simulink model "uas_main"  (R2021a)
settings: Solver=FixedStepAuto  StartTime=0.0  StopTime=5  FixedStep=sample_time  RelTol=1e-3
model workspace: external: MAT-File (data not in the file)
values from neighbouring files (symbols this model uses):
  arm_length = 0.17    [uas_parameters.m]    (also in uas_parameters.mat)
  drag_coefficient = 0.47    [uas_parameters.m]    (also in uas_parameters.mat)
  g = 9.80665    [uas_parameters.m]    (also in uas_parameters.mat)
  inertia_xx = 0.007    [uas_parameters.m]    (also in uas_parameters.mat)
  inertia_yy = 0.007    [uas_parameters.m]    (also in uas_parameters.mat)
  inertia_zz = 0.012    [uas_parameters.m]    (also in uas_parameters.mat)
  mass_drone = 0.68    [uas_parameters.m]    (also in uas_parameters.mat)
  mass_total = mass_drone + mass_rod + mass_tip    (= 0.68)    [uas_parameters.m]    (also in uas_parameters.mat)
  max_rot_velocity = 838    [uas_parameters.m]    (also in uas_parameters.mat)
  mix_matrix = inv(motor_constant * allocation_matrix)    [uas_parameters.m]    (also in uas_parameters.mat = [29244.6230836 29244.6230836 29244.6230836 29244.6230836 -5.)
  moment_constant = 0.016    [uas_parameters.m]    (also in uas_parameters.mat)
  motor_constant = 8.54858e-06    [uas_parameters.m]    (also in uas_parameters.mat)
  poly_traj = uas_minimum_snap(knots, order, waypoints, corridors, make_plots)    [uas_trajectory.m]
  publish_rate = 1 * sample_time    (= 0.04)    [uas_parameters.m]    (also in uas_parameters.mat)
  reference_area = pi * 75e-3^2    (= 0.0176714586764)    [uas_parameters.m]    (also in uas_parameters.mat)
  rotor_offset_top = 0.01    [uas_parameters.m]    (also in uas_parameters.mat)
  route = [0 0 1 ; 9 0 1 ; 9 5 1; 7 5 1; 7 7 1; 5 7 1; 5 5 1; 3 5 1]    [uas_parameters.m]    (also in uas_parameters.mat = [0  0  1; 9  0  1; 9  9  1])
  sample_time = 4e-2    (= 0.04)    [uas_parameters.m]    (also in uas_parameters.mat)
  x0 = 36    [uas_parameters.m]    (also in uas_parameters.mat)
  y0 = 80    [uas_parameters.m]    (also in uas_parameters.mat)
  z0 = 1    [uas_parameters.m]    (also in uas_parameters.mat)
undefined symbols (not defined in the file or in its folder): Angular, Linear, Pose, Position, quat2rotm, X, Y, Z
libraries: nesl_utility x32, sm_lib x25, robotlib x9, simulink x1, sim3dlib x1, uavsim3dlib x1, vrlib x1
(part 1 of 2)
settings Model: EnablePacing=on  Creator=david  LastModifiedBy=emilm
settings SolverCC: AlgebraicLoopSolver=TrustRegion
settings DataIOCC: LimitDataPoints=on  MaxDataPoints=10000
settings OptimizationCC: EnhancedBackFolding=on  PassReuseOutputArgsThreshold=0  ZeroExternalMemoryAtStartup=off  ZeroInternalMemoryAtStartup=off  MaxStackSize=64  OptimizeBlockOrder=speed  DifferentSizesBufferReuse=on  OptimizationCustomize=off
settings DebuggingCC: ParameterTunabilityLossMsg=error  AllowSymbolicDim=off  SFUnexpectedBacktrackingDiag=warning  SFNoUnconditionalDefaultTransitionDiag=warning  SFExecutionAtInitializationDiag=none  SFMachineParentedDataDiag=warning  UnderSpecifiedDimensionMsg=warning  ArithmeticOperatorsInVariantConditions=warning
settings HardwareCC: ProdBitPerPointer=32  ProdBitPerSizeT=32  ProdBitPerPtrDiffT=32  ProdLargestAtomicFloat=None  ProdIntDivRoundTo=Undefined  ProdEndianess=Unspecified  ProdWordSize=32  ProdHWDeviceType=Generic->Unspecified (assume 32-bit Generic)  UseEmbeddedCoderFeatures=off
settings SFSimCC: SimUseLocalCustomCode=off  MATLABDynamicMemAlloc=off  CustomCodeUndefinedFunction=UseInterfaceOnly  SimTargetLang=C++
settings RTWCC: SystemTargetFile=ert.tlc  HardwareBoard=Robot Operating System (ROS)  TLCOptions="-aInlineSetEventsForThisBaseRateFcn=TLC_FALSE -aSuppressMultiTaskScheduler=TLC_FALSE  -aRateBasedStepFcn=0"  TemplateMakefile=ert_default_tmf  RTWUseLocalCustomCode=off  Toolchain=Catkin  TargetLang=C++
settings CodeAppCC: ForceParamTrailComments=on  OperatorAnnotations=on
settings ERTTargetCC: ERTCustomFileBanners=off  CodeInterfacePackaging=C++ class  SupportContinuousTime=on  SupportNonInlinedSFcns=on  RemoveResetFunc=off  ModelStepFunctionPrototypeControlCompliant=off  RootIOFormat=Structure reference
settings ConfigComp: CovMetricSettings=dw  CovSaveCumulativeToWorkspaceVar=on  CovSaveSingleToWorkspaceVar=on  CovExternalEMLEnable=off  CovSFcnEnable=off
settings SimscapeCC: SimscapeLogType=all  SimscapeLogSimulationStatistics=on  SimscapeLogDataHistory=10000
settings ExplorerConfigSet: InternalSimMechanicsExplorerSettings="<ExplorerConfiguration><canonicalview>default</canonicalview><AnimationSetting><BasePlaybackSpeed>1.0</BasePlaybackSpeed><PlaybackSpeedFactor>1.0</PlaybackSpeedFactor></AnimationSetting><TilePanel><TileInfo><Tiles Columns=\"1\" Count=\"1\" Rows=\"1\"><Column Weight=\"1\"/><Row Weight=\"1\"/><Tile Height=\"1\" Width=\"1\" X=\"0\" Y=\"0\"/></Tiles></TileInfo><SceneInfo><SceneViewer><BGColor><R>0.400000005960464478</R><G>0.400000005960464478</G><B>0.400000005960464478</B></BGColor><Camera><DoPerspective>off</DoPerspective><Position><X>7.41918867546502359</X><Y>0.562842449888731333</Y><Z>8.36768126399918444</Z></Position><Center><X>4.24878770726833288</X><Y>4.27540210027623324</Y><Z>0.996100590645515815</Z></Center><Up><X>-0.578313069199200891</X><Y>0.601173295476169489</Y><Z>0.551493121262380703</Z></Up><ViewLimDist>1</ViewLimDist><YLim>5.48746925830841104</YLim><XLim>8.41878250057976274</XLim></Camera></SceneViewer></SceneInfo></TilePanel><MechEditorPanel><Cameras/><GfxPanelCameraMap/><VideoCreator><PlaybackSpeedRatio>1.0</PlaybackSpeedRatio><FrameRate>30</FrameRate><VideoFormat>Motion JPEG AVI</VideoFormat><FrameSize>auto</FrameSize></VideoCreator></MechEditorPanel></ExplorerConfiguration>"

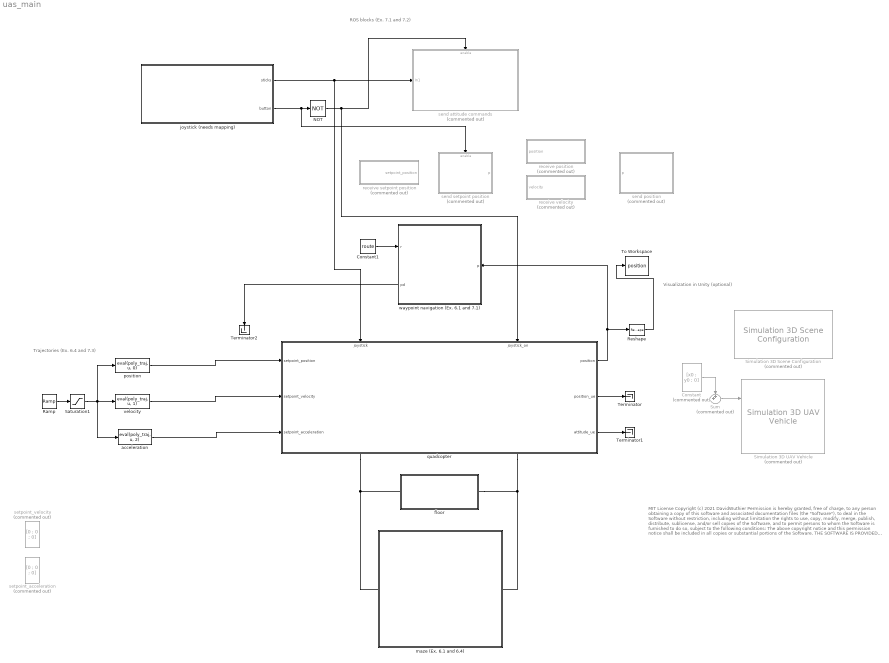
== system uas_main ==
  note: MIT License
      |
      | Copyright (c) 2021 DavidWuthier
      |
      | Permission is hereby granted, free of charge, to any person obtaining a copy
      | of this software and associated documentation files (the "Software"), to deal
      | in the Software without restriction, including without limitation the rights
      | to use, copy, modify, merge, publish, distribute, sublicense, and/or sell
      | copies of the Software, and to permit persons to whom the Software is
      | furnished to do so, subject to the following conditions:
      |
      | The above copyright notice and this permission notice shall be included in all
      | copies or substantial portions of the Software.
      |
      | THE SOFTWARE IS PROVIDED "AS IS", WITHOUT WARRANTY OF ANY KIND, EXPRESS OR
      | IMPLIED, INCLUDING BUT NOT LIMITED TO THE WARRANTIES OF MERCHANTABILITY,
      | FITNESS FOR A PARTICULAR PURPOSE AND NONINFRINGEMENT. IN NO EVENT SHALL THE
      | AUTHORS OR COPYRIGHT HOLDERS BE LIABLE FOR ANY CLAIM, DAMAGES OR OTHER
      | LIABILITY, WHETHER IN AN ACTION OF CONTRACT, TORT OR OTHERWISE, ARISING FROM,
      | OUT OF OR IN CONNECTION WITH THE SOFTWARE OR THE USE OR OTHER DEALINGS IN THE
      | SOFTWARE.
  note: Visualization in Unity (optional)
  note: Trajectories (Ex. 6.4 and 7.3)
  note: ROS blocks (Ex. 7.1 and 7.2)
  Constant : Constant  Commented=on  Value=[x0 ; y0 ; 0]  VectorParams1D=off
  Constant1 : Constant  Value=route
  NOT : Logic  Operator=NOT  IconShape=distinctive  AllPortsSameDT=off  OutDataTypeStr=boolean
  Ramp : simulink/Sources/Ramp  slope=1  start=0  InitialOutput=0
  Reshape : Reshape  OutputDimensions=[3,:]
  Saturation1 : Saturate  UpperLimit=knots(end)  LowerLimit=0
  Simulation 3D Scene Configuration : sim3dlib/Simulation 3D Scene Configuration  Priority=0  Commented=on  ProjectFormat=Default Scenes  SceneDesc=US city block  ProjectName=C:\Program Files\MATLAB\R2021a\toolbox\shared\sim3d_projects\automotive_project\UE4\WindowsNoEditor\VehicleSimulation.exe  ScenePath=/Game/Maps/USCityBlock  vehTagList={'Scene Origin';'SimulinkVehicle1'}  vehTag=SimulinkVehicle1  OpVisEn=off  Ts=sample_time  EnableWindow=on  EnableWeather=off  SunAltitude=40.0  SunAzimuth=90  clouds=10  wind=1  fog=0  rain=0  sensorTag=MainCamera1  sensorId=1  sensorName=MainCamera1  mountLoc=Origin  offsetFlag=off  tmountOffset=[0, 0, 0]  rmountOffset=[0, 0, 0]  HorizontalResolution=1280  VerticalResolution=720  HorizontalFOV=60  mountPoint=[0 0 0]  mountOrientation=[0 0 0]  aMode=4  ID=1
      settings: SourceProductBaseCode=DR,UV,VE
  Simulation 3D UAV Vehicle : uavsim3dlib/Simulation 3D UAV Vehicle  Commented=on  Mesh=Quadrotor  Color=Black  ActorName=SimulinkVehicle1  InitialTranslation=[x0 y0 z0]  InitialRotation=[0 0 0]  SampleTime=-1  ActorType=SimulinkVehicle  ID=1  aMode=4  ActorTag=SimulinkVehicle1
      settings: SourceProductBaseCode=UV
  Sum : Sum  Commented=on  Inputs=++|
  Terminator : Terminator
  Terminator1 : Terminator
  Terminator2 : Terminator
  To Workspace : ToWorkspace  VariableName=position  SampleTime=-1
  acceleration : MATLABFcn  MATLABFcn=eval(poly_traj, u, 2)  OutputDimensions=[3 1]  Output1D=off
  floor : Subsystem
  joystick (needs mapping) : Subsystem
  maze (Ex. 6.1 and 6.4) : Subsystem
      mask Display: image('$imagefile'); % Use "Edit Image" on toolstrip to change.
  position : MATLABFcn  MATLABFcn=eval(poly_traj, u, 0)  OutputDimensions=[3 1]  Output1D=off
  quadcopter : Subsystem
      settings: PortSchema="{\"entries\":[{\"content\":{\"sides\":[{\"content\":{\"connectorIds\":[\"In1\",\"In2\",\"In3\"]},\"type\":\"ConnectorPlacement.EquallySpacedRectSide\",\"uuid\":\"ed16c4a7-5f5f-48d5-8471-b227eef37b0b\"},{\"content\":{\"connectorIds\":[\"Out1\",\"Out2\",\"Out3\"],\"side\":\"RIGHT\"},\"type\":\"ConnectorPlacement.EquallySpacedRectSide\",\"uuid\":\"303ea24f-0a15-469a-b5d8-cc8b33d29b5f\"},{\"content\":{\"connectorIds\":[\"In4\",\"In5\"],\"side\":\"TOP\"},\"type\":\"ConnectorPlacement.EquallySpacedRectSide\",\"uuid\":\"d3970502-0872-434b-b7c5-387e72ad4178\"},{\"content\":{\"connectorIds\":[\"RConn1\",\"RConn2\"],\"side\":\"BOTTOM\"},\"type\":\"ConnectorPlacement.EquallySpacedRectSide\",\"uuid\":\"dd808c8e-2f91-44fb-8d51-5dec3bd81dd9\"}]},\"type\":\"ConnectorPlacement.EquallySpacedConnector\",\"uuid\":\"aacf4a84-08b7-4fd3-a02a-51c4e2a4df71\"}],\"packageUris\":[\"http://schema.mathworks.com/mf0/Connector/R2020b\"],\"version\":\"1.0\"}"
  receive position : Subsystem  Commented=on
  receive setpoint position : Subsystem  Commented=on
  receive velocity : Subsystem  Commented=on
  send attitude commands : Subsystem  Commented=on
  send position : Subsystem  Commented=on
  send setpoint position : Subsystem  Commented=on
  setpoint_acceleration : Constant  Commented=on  Value=[0 ; 0 ; 0]  VectorParams1D=off
  setpoint_velocity : Constant  Commented=on  Value=[0 ; 0 ; 0]  VectorParams1D=off
  velocity : MATLABFcn  MATLABFcn=eval(poly_traj, u, 1)  OutputDimensions=[3 1]  Output1D=off
  waypoint navigation (Ex. 6.1 and 7.1) : Stateflow chart  TreatAsAtomicUnit=on
      settings: PortSchema="{\"entries\":[{\"content\":{\"sides\":[{\"content\":{\"connectorIds\":[\"In1\",\"Out1\"]},\"type\":\"ConnectorPlacement.EquallySpacedRectSide\",\"uuid\":\"7c2fff0d-1179-4786-9432-1971d7acd904\"},{\"content\":{\"connectorIds\":[\"In2\"],\"side\":\"RIGHT\"},\"type\":\"ConnectorPlacement.EquallySpacedRectSide\",\"uuid\":\"377a8206-b310-41c0-9a17-faf5318c89cb\"},{\"content\":{\"connectorIds\":[],\"side\":\"TOP\"},\"type\":\"ConnectorPlacement.EquallySpacedRectSide\",\"uuid\":\"b953090a-ffdb-4e30-a5fe-7bef9655f1cf\"},{\"content\":{\"connectorIds\":[],\"side\":\"BOTTOM\"},\"type\":\"ConnectorPlacement.EquallySpacedRectSide\",\"uuid\":\"03dc7a24-529e-4020-b953-d1c4751c5c80\"}]},\"type\":\"ConnectorPlacement.EquallySpacedConnector\",\"uuid\":\"03bac9f4-6480-492d-9af3-57aec4db8fd8\"}],\"packageUris\":[\"http://schema.mathworks.com/mf0/Connector/R2020b\"],\"version\":\"1.0\"}"
  wires:
  Sum/1 -> Simulation 3D UAV Vehicle/1
  Constant/1 -> Sum/1
  Constant1/1 -> waypoint navigation (Ex. 6.1 and 7.1)/1(r)
  Saturation1/1 -> acceleration/1, position/1, velocity/1
  Ramp/1 -> Saturation1/1
  NOT/1 -> quadcopter/5(joystick_on), send attitude commands/Enable
  joystick (needs mapping)/1(sticks) -> send attitude commands/1(In1), quadcopter/4(joystick)
  joystick (needs mapping)/2(button) -> NOT/1, send setpoint position/Enable
  quadcopter/1(position) -> Reshape/1, waypoint navigation (Ex. 6.1 and 7.1)/2(p)
  quadcopter/2(position_ue) -> Terminator/1
  quadcopter/3(attitude_ue) -> Terminator1/1
  Reshape/1 -> To Workspace/1
  waypoint navigation (Ex. 6.1 and 7.1)/1(pd) -> Terminator2/1
  position/1 -> quadcopter/1(setpoint_position)
  velocity/1 -> quadcopter/2(setpoint_velocity)
  acceleration/1 -> quadcopter/3(setpoint_acceleration)
  connections:
  floor/LConn1 -- quadcopter/RConn1 -- maze (Ex. 6.1 and 6.4)/LConn1
  floor/RConn1 -- quadcopter/RConn2 -- maze (Ex. 6.1 and 6.4)/RConn1

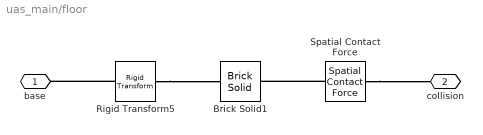
== system uas_main/floor ==
  Brick Solid1 : sm_lib/Body Elements/Brick Solid  GraphicAmbientColor=[0.15 0.15 0.15 1.0]  BasedOnType=Density  BrickDimensions=[3 3 0.1]  BrickDimensionUnits=m  CenterOfMass=[0 0 0]  CenterOfMassUnits=m  GraphicDiffuseColor=[0.4 0.4 0.4]  Density=0  DensityUnits=kg/m^3  DoExposeReferenceFrame=on  GraphicEmissiveColor=[0.0 0.0 0.0 1.0]  ExportEntireGeometry=on  SerializedFrames=<Frames/>  MarkerShape=Sphere  MarkerSize=10  GraphicType=FromGeometry  InertiaType=CalculateFromGeometry  Mass=1  MassUnits=kg  MomentsOfInertia=[1 1 1]  MomentsOfInertiaUnits=kg*m^2  GraphicOpacity=1  ProductsOfInertia=[0 0 0]  ProductsOfInertiaUnits=kg*m^2  GraphicShininess=75  GraphicSpecularColor=[0.5 0.5 0.5 1.0]  GraphicVisPropType=SimpleVisualProperties
  Rigid Transform5 : sm_lib/Frames and Transforms/Rigid Transform  TranslationMethod=StandardAxis  TranslationStandardOffset=0.05  TranslationLengthUnit=m  TranslationStandardAxis=-Z  TranslationCartesianOffset=[0 0 0]  TranslationROffset=0  TranslationROffsetUnits=m  TranslationZOffset=0  TranslationZOffsetUnits=m  TranslationThetaOffset=0  TranslationThetaOffsetUnits=deg  RotationMethod=None  RotationAngleUnits=deg  RotationStandardAxis=+Z  RotationAngle=0.0  RotationArbitraryAxis=[0 0 1]  FollAlignAxisA=+X  BaseAlignAxisA=+Y  FollAlignAxisB=+Y  BaseAlignAxisB=+Z  RotationSequenceAxes=FollowerAxes  RotationSequence=XYX  RotationSequenceAngles=[0 0 0]  RotationSequenceAnglesUnits=deg  RotationMatrix=[1 0 0; 0 1 0; 0 0 1]
  Spatial Contact Force : sm_lib/Forces and Torques/Spatial Contact Force  CoefficientOfDynamicFriction=0.3  CoefficientOfStaticFriction=0.5  SenseContactBaseRotation=off  SenseContactBaseTranslation=off  NormalDamping=critical_damping_wall  NormalDampingUnits=N/(m/s)  SenseContactFollowerRotation=off  SenseContactFollowerTranslation=off  SenseContactSignal=off  NormalStiffness=stiffness_wall  NormalStiffnessUnits=N/m  FrictionalCriticalVelocity=1e-3  FrictionalCriticalVelocityUnits=m/s  ZeroCrossDetectContactStartAndEnd=off  FrictionType=SmoothStickSlip  SenseFrictionalForceMagnitude=off  SenseNormalForceMagnitude=off  NormalForceType=SmoothSpringDamper  SenseNormalVelocity=off  SenseSeparationDistance=off  SenseTangentialVelocity=off  SenseTangentialVelocityMagnitude=off  NormalTransitionRegionWidth=1e-4  NormalTransitionRegionWidthUnits=m
  base : PMIOPort  Side=Left
  collision : PMIOPort  Port=2  Side=Right
  connections:
  Rigid Transform5/RConn1 -- Brick Solid1/RConn1
  Rigid Transform5/LConn1 -- base/RConn1
  Spatial Contact Force/RConn1 -- Brick Solid1/LConn1
  Spatial Contact Force/LConn1 -- collision/RConn1

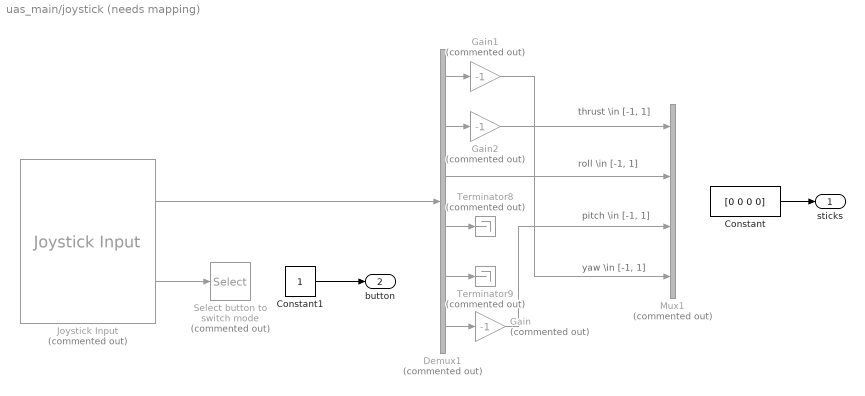
== system uas_main/joystick (needs mapping) ==
  note: thrust \in [-1, 1]
  note: roll \in [-1, 1]
  note: pitch \in [-1, 1]
  note: yaw \in [-1, 1]
  Constant : Constant  Value=[0 0 0 0]
  Constant1 : Constant
  Demux1 : Demux  Commented=on  Outputs=6
  Gain : Gain  Commented=on  Gain=-1
  Gain1 : Gain  Commented=on  Gain=-1
  Gain2 : Gain  Commented=on  Gain=-1
  Joystick Input : vrlib/Joystick Input  Commented=on  joyid=1  adjustports=on  forcefeed=off
  Mux1 : Mux  Commented=on
  Select button to switch mode : Selector  Commented=on  InputPortWidth=15  IndexOptions=Index vector (dialog)  Indices=8  OutputSizes=1
  Terminator8 : Terminator  Commented=on
  Terminator9 : Terminator  Commented=on
  sticks : Outport
  button : Outport  Port=2
  wires:
  Gain1/1 -> Mux1/4
  Joystick Input/1 -> Demux1/1
  Gain2/1 -> Mux1/1
  Demux1/1 -> Gain1/1
  Joystick Input/2 -> Select button to switch mode/1
  Demux1/6 -> Gain/1
  Demux1/5 -> Terminator9/1
  Demux1/3 -> Mux1/2
  Demux1/2 -> Gain2/1
  Demux1/4 -> Terminator8/1
  Gain/1 -> Mux1/3
  Constant/1 -> sticks/1
  Constant1/1 -> button/1

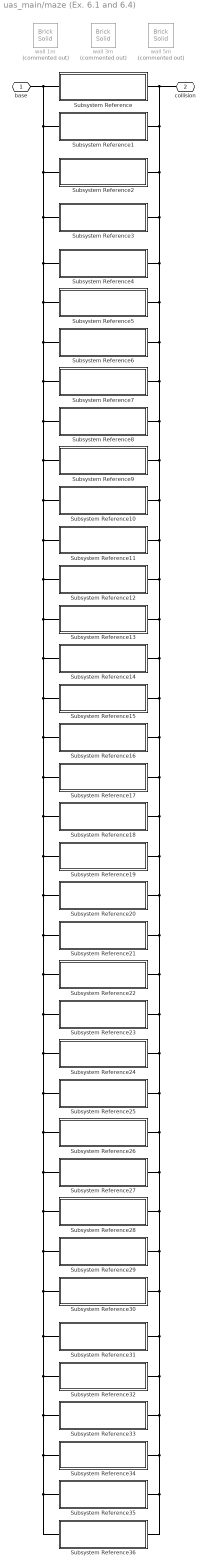
== system uas_main/maze (Ex. 6.1 and 6.4) ==
  Subsystem Reference : Subsystem  ReferencedSubsystem=uas_wall  l=5  x=-1  y=1.5  yaw=0
  Subsystem Reference1 : Subsystem  ReferencedSubsystem=uas_wall  l=5  x=-1  y=7.5  yaw=0
  Subsystem Reference10 : Subsystem  ReferencedSubsystem=uas_wall  l=5  x=7.5  y=10  yaw=pi/2
  Subsystem Reference11 : Subsystem  ReferencedSubsystem=uas_wall  l=5  x=5  y=10  yaw=pi/2
  Subsystem Reference12 : Subsystem  ReferencedSubsystem=uas_wall  l=5  x=1.5  y=1  yaw=pi/2
  Subsystem Reference13 : Subsystem  ReferencedSubsystem=uas_wall  l=3  x=4.5  y=1  yaw=pi/2
  Subsystem Reference14 : Subsystem  ReferencedSubsystem=uas_wall  l=3  x=8  y=2.5  yaw=0
  Subsystem Reference15 : Subsystem  ReferencedSubsystem=uas_wall  l=1  x=6  y=4.5  yaw=0
  Subsystem Reference16 : Subsystem  ReferencedSubsystem=uas_wall  l=1  x=6  y=1.5  yaw=0
  Subsystem Reference17 : Subsystem  ReferencedSubsystem=uas_wall  l=1  x=2  y=1.5  yaw=0
  Subsystem Reference18 : Subsystem  ReferencedSubsystem=uas_wall  l=1  x=0  y=2.5  yaw=0
  Subsystem Reference19 : Subsystem  ReferencedSubsystem=uas_wall  l=5  x=5.5  y=4  yaw=pi/2
  Subsystem Reference2 : Subsystem  ReferencedSubsystem=uas_wall  l=5  x=-1  y=5  yaw=0
  Subsystem Reference20 : Subsystem  ReferencedSubsystem=uas_wall  l=1  x=4  y=3.5  yaw=0
  Subsystem Reference21 : Subsystem  ReferencedSubsystem=uas_wall  l=1  x=2.5  y=4  yaw=pi/2
  Subsystem Reference22 : Subsystem  ReferencedSubsystem=uas_wall  l=1  x=0.5  y=2  yaw=pi/2
  Subsystem Reference23 : Subsystem  ReferencedSubsystem=uas_wall  l=1  x=1.5  y=2  yaw=pi/2
  Subsystem Reference24 : Subsystem  ReferencedSubsystem=uas_wall  l=1  x=-0.5  y=3  yaw=pi/2
  Subsystem Reference25 : Subsystem  ReferencedSubsystem=uas_wall  l=1  x=2  y=4.5  yaw=0
  Subsystem Reference26 : Subsystem  ReferencedSubsystem=uas_wall  l=1  x=1.5  y=5  yaw=pi/2
  Subsystem Reference27 : Subsystem  ReferencedSubsystem=uas_wall  l=1  x=0.5  y=7  yaw=pi/2
  Subsystem Reference28 : Subsystem  ReferencedSubsystem=uas_wall  l=1  x=1  y=7.5  yaw=0
  Subsystem Reference29 : Subsystem  ReferencedSubsystem=uas_wall  l=2  x=8  y=7  yaw=0
  Subsystem Reference3 : Subsystem  ReferencedSubsystem=uas_wall  l=5  x=10  y=1.5  yaw=0
  Subsystem Reference30 : Subsystem  ReferencedSubsystem=uas_wall  l=1  x=-0.5  y=7  yaw=pi/2
  Subsystem Reference31 : Subsystem  ReferencedSubsystem=uas_wall  l=1  x=6  y=5.5  yaw=0
  Subsystem Reference32 : Subsystem  ReferencedSubsystem=uas_wall  l=5  x=5.5  y=8  yaw=pi/2
  Subsystem Reference33 : Subsystem  ReferencedSubsystem=uas_wall  l=1  x=3.5  y=7  yaw=pi/2
  Subsystem Reference34 : Subsystem  ReferencedSubsystem=uas_wall  l=1  x=3  y=7.5  yaw=0
  Subsystem Reference35 : Subsystem  ReferencedSubsystem=uas_wall  l=1  x=4  y=6.5  yaw=0
  Subsystem Reference36 : Subsystem  ReferencedSubsystem=uas_wall  l=1  x=4  y=7.5  yaw=0
  Subsystem Reference4 : Subsystem  ReferencedSubsystem=uas_wall  l=5  x=10  y=7.5  yaw=0
  Subsystem Reference5 : Subsystem  ReferencedSubsystem=uas_wall  l=5  x=10  y=5  yaw=0
  Subsystem Reference6 : Subsystem  ReferencedSubsystem=uas_wall  l=5  x=1.5  y=-1  yaw=pi/2
  Subsystem Reference7 : Subsystem  ReferencedSubsystem=uas_wall  l=5  x=7.5  y=-1  yaw=pi/2
  Subsystem Reference8 : Subsystem  ReferencedSubsystem=uas_wall  l=5  x=5  y=-1  yaw=pi/2
  Subsystem Reference9 : Subsystem  ReferencedSubsystem=uas_wall  l=5  x=1.5  y=10  yaw=pi/2
  wall 1m : sm_lib/Body Elements/Brick Solid  Commented=on  GraphicAmbientColor=[0.15 0.15 0.15 1.0]  BasedOnType=Density  BrickDimensions=[0.1 1 2]  BrickDimensionUnits=m  CenterOfMass=[0 0 0]  CenterOfMassUnits=m  GraphicDiffuseColor=wall_color  Density=1000  DensityUnits=kg/m^3  DoExposeReferenceFrame=on  GraphicEmissiveColor=[0.0 0.0 0.0 1.0]  ExportEntireGeometry=on  SerializedFrames=<Frames/>  MarkerShape=Sphere  MarkerSize=10  GraphicType=FromGeometry  InertiaType=CalculateFromGeometry  Mass=1  MassUnits=kg  MomentsOfInertia=[1 1 1]  MomentsOfInertiaUnits=kg*m^2  GraphicOpacity=1.0  ProductsOfInertia=[0 0 0]  ProductsOfInertiaUnits=kg*m^2  GraphicShininess=75  GraphicSpecularColor=[0.5 0.5 0.5 1.0]  GraphicVisPropType=SimpleVisualProperties
  wall 3m : sm_lib/Body Elements/Brick Solid  Commented=on  GraphicAmbientColor=[0.15 0.15 0.15 1.0]  BasedOnType=Density  BrickDimensions=[0.1 3 2]  BrickDimensionUnits=m  CenterOfMass=[0 0 0]  CenterOfMassUnits=m  GraphicDiffuseColor=wall_color  Density=1000  DensityUnits=kg/m^3  DoExposeReferenceFrame=on  GraphicEmissiveColor=[0.0 0.0 0.0 1.0]  ExportEntireGeometry=on  SerializedFrames=<Frames/>  MarkerShape=Sphere  MarkerSize=10  GraphicType=FromGeometry  InertiaType=CalculateFromGeometry  Mass=1  MassUnits=kg  MomentsOfInertia=[1 1 1]  MomentsOfInertiaUnits=kg*m^2  GraphicOpacity=1.0  ProductsOfInertia=[0 0 0]  ProductsOfInertiaUnits=kg*m^2  GraphicShininess=75  GraphicSpecularColor=[0.5 0.5 0.5 1.0]  GraphicVisPropType=SimpleVisualProperties
  wall 5m : sm_lib/Body Elements/Brick Solid  Commented=on  GraphicAmbientColor=[0.15 0.15 0.15 1.0]  BasedOnType=Density  BrickDimensions=[0.1 5 2]  BrickDimensionUnits=m  CenterOfMass=[0 0 0]  CenterOfMassUnits=m  GraphicDiffuseColor=wall_color  Density=1000  DensityUnits=kg/m^3  DoExposeReferenceFrame=on  GraphicEmissiveColor=[0.0 0.0 0.0 1.0]  ExportEntireGeometry=on  SerializedFrames=<Frames/>  MarkerShape=Sphere  MarkerSize=10  GraphicType=FromGeometry  InertiaType=CalculateFromGeometry  Mass=1  MassUnits=kg  MomentsOfInertia=[1 1 1]  MomentsOfInertiaUnits=kg*m^2  GraphicOpacity=1.0  ProductsOfInertia=[0 0 0]  ProductsOfInertiaUnits=kg*m^2  GraphicShininess=75  GraphicSpecularColor=[0.5 0.5 0.5 1.0]  GraphicVisPropType=SimpleVisualProperties
  base : PMIOPort  Side=Left
  collision : PMIOPort  Port=2  Side=Right
  connections:
  Subsystem Reference35/LConn1 -- Subsystem Reference36/LConn1 -- base/RConn1 -- Subsystem Reference/LConn1 -- Subsystem Reference1/LConn1 -- Subsystem Reference2/LConn1 -- Subsystem Reference3/LConn1 -- Subsystem Reference4/LConn1 -- Subsystem Reference5/LConn1 -- Subsystem Reference6/LConn1 -- Subsystem Reference7/LConn1 -- Subsystem Reference8/LConn1 -- Subsystem Reference9/LConn1 -- Subsystem Reference10/LConn1 -- Subsystem Reference11/LConn1 -- Subsystem Reference12/LConn1 -- Subsystem Reference13/LConn1 -- Subsystem Reference14/LConn1 -- Subsystem Reference15/LConn1 -- Subsystem Reference16/LConn1 -- Subsystem Reference17/LConn1 -- Subsystem Reference18/LConn1 -- Subsystem Reference19/LConn1 -- Subsystem Reference20/LConn1 -- Subsystem Reference21/LConn1 -- Subsystem Reference22/LConn1 -- Subsystem Reference23/LConn1 -- Subsystem Reference24/LConn1 -- Subsystem Reference25/LConn1 -- Subsystem Reference26/LConn1 -- Subsystem Reference27/LConn1 -- Subsystem Reference28/LConn1 -- Subsystem Reference29/LConn1 -- Subsystem Reference30/LConn1 -- Subsystem Reference31/LConn1 -- Subsystem Reference32/LConn1 -- Subsystem Reference33/LConn1 -- Subsystem Reference34/LConn1
  Subsystem Reference32/RConn1 -- Subsystem Reference36/RConn1 -- Subsystem Reference35/RConn1 -- Subsystem Reference34/RConn1 -- Subsystem Reference33/RConn1 -- collision/RConn1 -- Subsystem Reference/RConn1 -- Subsystem Reference1/RConn1 -- Subsystem Reference2/RConn1 -- Subsystem Reference3/RConn1 -- Subsystem Reference4/RConn1 -- Subsystem Reference5/RConn1 -- Subsystem Reference6/RConn1 -- Subsystem Reference7/RConn1 -- Subsystem Reference8/RConn1 -- Subsystem Reference9/RConn1 -- Subsystem Reference10/RConn1 -- Subsystem Reference11/RConn1 -- Subsystem Reference12/RConn1 -- Subsystem Reference13/RConn1 -- Subsystem Reference14/RConn1 -- Subsystem Reference15/RConn1 -- Subsystem Reference16/RConn1 -- Subsystem Reference17/RConn1 -- Subsystem Reference18/RConn1 -- Subsystem Reference19/RConn1 -- Subsystem Reference20/RConn1 -- Subsystem Reference21/RConn1 -- Subsystem Reference22/RConn1 -- Subsystem Reference23/RConn1 -- Subsystem Reference24/RConn1 -- Subsystem Reference25/RConn1 -- Subsystem Reference26/RConn1 -- Subsystem Reference27/RConn1 -- Subsystem Reference28/RConn1 -- Subsystem Reference29/RConn1 -- Subsystem Reference30/RConn1 -- Subsystem Reference31/RConn1

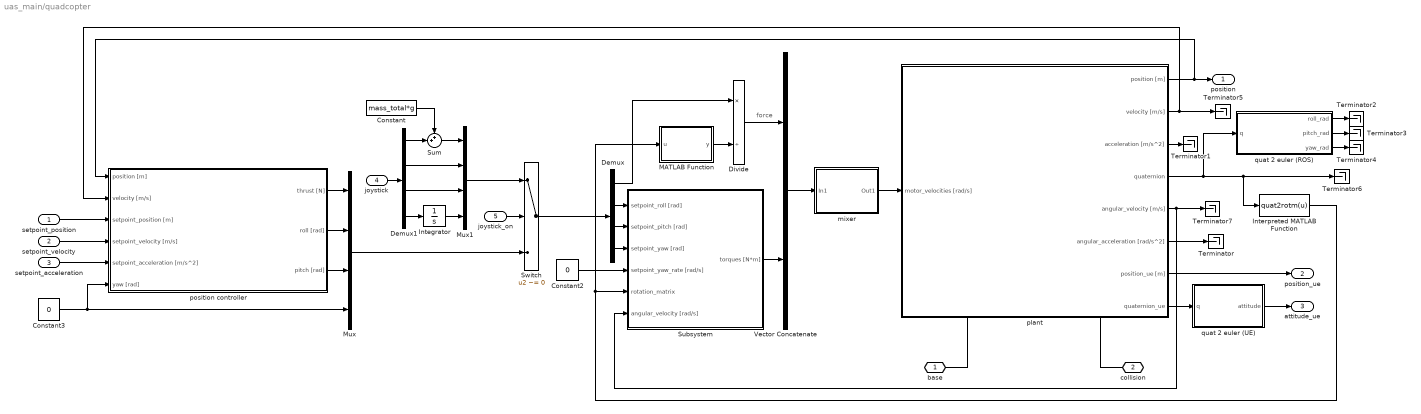
== system uas_main/quadcopter ==
  note: force
  setpoint_position : Inport
  setpoint_velocity : Inport  Port=2
  setpoint_acceleration : Inport  Port=3
  joystick : Inport  Port=4
  joystick_on : Inport  Port=5
  Constant : Constant  Value=mass_total*g
  Constant2 : Constant  Value=0
  Constant3 : Constant  Value=0
  Demux : Demux
  Demux1 : Demux
  Divide : Product  Inputs=*/
  Integrator : Integrator  WrapState=on
  Interpreted MATLAB Function : MATLABFcn  MATLABFcn=quat2rotm(u)  Output1D=off
  MATLAB Function : MATLAB Function  TreatAsAtomicUnit=on
  Mux : Mux
  Mux1 : Mux
  Subsystem : Subsystem
      mask Display: image('$imagefile'); % Use "Edit Image" on toolstrip to change.
  Sum : Sum  Inputs=++|
  Switch : Switch  Criteria=u2 ~= 0
  Terminator{,1..7} (8 alike) : Terminator
  Vector Concatenate : Concatenate
  mixer : Subsystem
  plant : Subsystem
      settings: PortSchema="{\"entries\":[{\"content\":{\"sides\":[{\"content\":{\"connectorIds\":[\"In1\"]},\"type\":\"ConnectorPlacement.EquallySpacedRectSide\",\"uuid\":\"6e9c785b-7a58-4a83-84e6-bbea81e0823c\"},{\"content\":{\"connectorIds\":[\"Out1\",\"Out2\",\"Out3\",\"Out4\",\"Out5\",\"Out6\",\"Out7\",\"Out8\"],\"side\":\"RIGHT\"},\"type\":\"ConnectorPlacement.EquallySpacedRectSide\",\"uuid\":\"b008e1e2-aa95-4897-b360-2fe655e93601\"},{\"content\":{\"connectorIds\":[],\"side\":\"TOP\"},\"type\":\"ConnectorPlacement.EquallySpacedRectSide\",\"uuid\":\"363cdb01-a5e5-4a3c-bce9-213e2ffac7b5\"},{\"content\":{\"connectorIds\":[\"RConn1\",\"RConn2\"],\"side\":\"BOTTOM\"},\"type\":\"ConnectorPlacement.EquallySpacedRectSide\",\"uuid\":\"8e0d8754-e9ec-4386-98a0-719833eb7e87\"}]},\"type\":\"ConnectorPlacement.EquallySpacedConnector\",\"uuid\":\"eb300e37-0abf-4331-8664-ac63688da223\"}],\"packageUris\":[\"http://schema.mathworks.com/mf0/Connector/R2020b\"],\"version\":\"1.0\"}"
      mask Display: image('$imagefile'); % Use "Edit Image" on toolstrip to change.
  position controller : Subsystem
      mask Display: image('$imagefile'); % Use "Edit Image" on toolstrip to change.
  quat 2 euler (ROS) : MATLAB Function  TreatAsAtomicUnit=on
  quat 2 euler (UE) : MATLAB Function  TreatAsAtomicUnit=on
  base : PMIOPort  Side=Right
  collision : PMIOPort  Port=2  Side=Right
  position : Outport
  position_ue : Outport  Port=2
  attitude_ue : Outport  Port=3
  wires:
  plant/4(quaternion) -> quat 2 euler (ROS)/1(q), Terminator6/1, Interpreted MATLAB Function/1
  plant/6(angular_acceleration [rad/s^2]) -> Terminator/1
  plant/3(acceleration [m/s^2]) -> Terminator1/1
  Interpreted MATLAB Function/1 -> MATLAB Function/1(u), Subsystem/5(rotation_matrix)
  plant/5(angular_velocity [m/s]) -> Terminator7/1, Subsystem/6(angular_velocity [rad/s])
  quat 2 euler (UE)/1(attitude) -> attitude_ue/1
  plant/8(quaternion_ue) -> quat 2 euler (UE)/1(q)
  plant/7(position_ue [m]) -> position_ue/1
  plant/2(velocity [m/s]) -> Terminator5/1, position controller/2(velocity [m/s])
  plant/1(position [m]) -> position controller/1(position [m]), position/1
  Constant2/1 -> Subsystem/4(setpoint_yaw_rate [rad/s])
  setpoint_acceleration/1 -> position controller/5(setpoint_acceleration [m/s^2])
  setpoint_velocity/1 -> position controller/4(setpoint_velocity [m/s])
  setpoint_position/1 -> position controller/3(setpoint_position [m])
  Constant3/1 -> Mux/4, position controller/6(yaw [rad])
  quat 2 euler (ROS)/1(roll_rad) -> Terminator2/1
  quat 2 euler (ROS)/2(pitch_rad) -> Terminator3/1
  quat 2 euler (ROS)/3(yaw_rad) -> Terminator4/1
  position controller/1(thrust [N]) -> Mux/1
  position controller/2(roll [rad]) -> Mux/2
  position controller/3(pitch [rad]) -> Mux/3
  Demux/2 -> Subsystem/1(setpoint_roll [rad])
  Demux/3 -> Subsystem/2(setpoint_pitch [rad])
  Demux/4 -> Subsystem/3(setpoint_yaw [rad])
  Switch/1 -> Demux/1
  Mux/1 -> Switch/3
  joystick_on/1 -> Switch/2
  joystick/1 -> Demux1/1
  Demux1/2 -> Mux1/2
  Demux1/3 -> Mux1/3
  Mux1/1 -> Switch/1
  Demux1/4 -> Integrator/1
  Integrator/1 -> Mux1/4
  Sum/1 -> Mux1/1
  Constant/1 -> Sum/1
  Demux1/1 -> Sum/2
  Demux/1 -> Divide/1
  Divide/1 -> Vector Concatenate/1
  Subsystem/1(torques [N*m]) -> Vector Concatenate/2
  MATLAB Function/1(y) -> Divide/2
  Vector Concatenate/1 -> mixer/1(In1)
  mixer/1(Out1) -> plant/1(motor_velocities [rad/s])
  connections:
  plant/RConn1 -- base/RConn1
  collision/RConn1 -- plant/RConn2

== system uas_main/receive position ==
  Bus Selector : BusSelector  OutputSignals=Pose.Position.X,Pose.Position.Y,Pose.Position.Z
  Mux : Mux  Inputs=3
  Subscribe : robotlib/Subscribe  topicSource=Select from ROS network  topic=/crazyflie/pose  messageType=geometry_msgs/PoseStamped  SampleTime=-1  legacyBusStruct=off  messageQueueLength=1
  Terminator5 : Terminator
  position : Outport
  wires:
  Subscribe/2 -> Bus Selector/1
  Mux/1 -> position/1
  Bus Selector/3 -> Mux/3  "<Z>"
  Bus Selector/1 -> Mux/1  "<X>"
  Bus Selector/2 -> Mux/2  "<Y>"
  Subscribe/1 -> Terminator5/1

== system uas_main/receive setpoint position ==
  Bus Selector : BusSelector  OutputSignals=Position.X,Position.Y,Position.Z
  Mux : Mux  Inputs=3
  Subscribe : robotlib/Subscribe  topicSource=Specify your own  topic=/crazyflie/cmd_position  messageType=geometry_msgs/Pose  SampleTime=-1  legacyBusStruct=off  messageQueueLength=1
  Terminator5 : Terminator
  setpoint_position : Outport
  wires:
  Subscribe/2 -> Bus Selector/1
  Mux/1 -> setpoint_position/1
  Bus Selector/3 -> Mux/3  "<Z>"
  Bus Selector/1 -> Mux/1  "<X>"
  Bus Selector/2 -> Mux/2  "<Y>"
  Subscribe/1 -> Terminator5/1

== system uas_main/receive velocity ==
  Bus Selector : BusSelector  OutputSignals=Twist.Linear.X,Twist.Linear.Y,Twist.Linear.Z
  Mux : Mux  Inputs=3
  Subscribe : robotlib/Subscribe  topicSource=Specify your own  topic=/crazyflie/twist  messageType=geometry_msgs/TwistStamped  SampleTime=-1  legacyBusStruct=off  messageQueueLength=1
  Terminator5 : Terminator
  velocity : Outport
  wires:
  Subscribe/2 -> Bus Selector/1
  Mux/1 -> velocity/1
  Bus Selector/3 -> Mux/3  "<Z>"
  Bus Selector/1 -> Mux/1  "<X>"
  Bus Selector/2 -> Mux/2  "<Y>"
  Subscribe/1 -> Terminator5/1

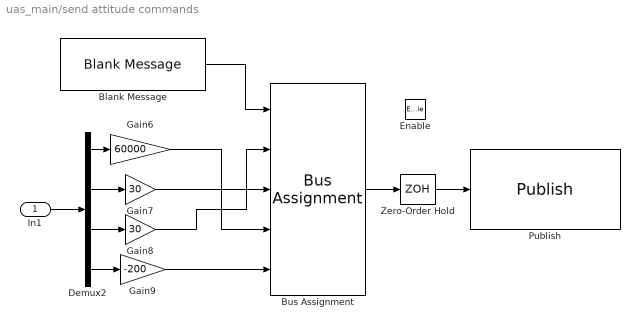
== system uas_main/send attitude commands ==
  In1 : Inport
  Enable : EnablePort
  Blank Message : robotlib/Blank Message  messageClass=Message  entityType=geometry_msgs/Twist  messageType=geometry_msgs/Twist  SampleTime=inf  legacyBusStruct=off
  Bus Assignment : BusAssignment  AssignedSignals=Linear.X,Linear.Y,Linear.Z,Angular.Z
  Demux2 : Demux
  Gain6 : Gain  Gain=60000
  Gain7 : Gain  Gain=30
  Gain8 : Gain  Gain=30
  Gain9 : Gain  Gain=-200
  Publish : robotlib/Publish  topicSource=Select from ROS network  topic=/crazyflie/cmd_vel  messageType=geometry_msgs/Twist  legacyBusStruct=off  messageQueueLength=1
  Zero-Order Hold : ZeroOrderHold  SampleTime=1/25
  wires:
  Zero-Order Hold/1 -> Publish/1
  Blank Message/1 -> Bus Assignment/1
  Bus Assignment/1 -> Zero-Order Hold/1
  In1/1 -> Demux2/1
  Demux2/1 -> Gain6/1
  Demux2/2 -> Gain7/1
  Demux2/3 -> Gain8/1
  Demux2/4 -> Gain9/1
  Gain6/1 -> Bus Assignment/4
  Gain7/1 -> Bus Assignment/3
  Gain8/1 -> Bus Assignment/2
  Gain9/1 -> Bus Assignment/5

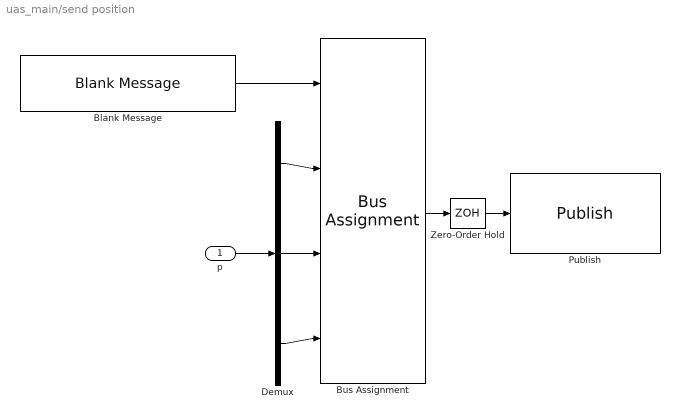
== system uas_main/send position ==
  p : Inport
  Blank Message : robotlib/Blank Message  messageClass=Message  entityType=geometry_msgs/PoseStamped  messageType=geometry_msgs/PoseStamped  SampleTime=inf  legacyBusStruct=off
  Bus Assignment : BusAssignment  AssignedSignals=Pose.Position.X,Pose.Position.Y,Pose.Position.Z
  Demux : Demux  Outputs=3
  Publish : robotlib/Publish  topicSource=Specify your own  topic=/crazyflie/pose  messageType=geometry_msgs/PoseStamped  legacyBusStruct=off  messageQueueLength=1
  Zero-Order Hold : ZeroOrderHold  SampleTime=publish_rate
  wires:
  Bus Assignment/1 -> Zero-Order Hold/1
  Blank Message/1 -> Bus Assignment/1
  Zero-Order Hold/1 -> Publish/1
  Demux/1 -> Bus Assignment/2
  Demux/2 -> Bus Assignment/3
  Demux/3 -> Bus Assignment/4
  p/1 -> Demux/1

== system uas_main/send setpoint position ==
  p : Inport
  Enable : EnablePort
  send setpoint position : Subsystem
  wires:
  p/1 -> send setpoint position/1(p)

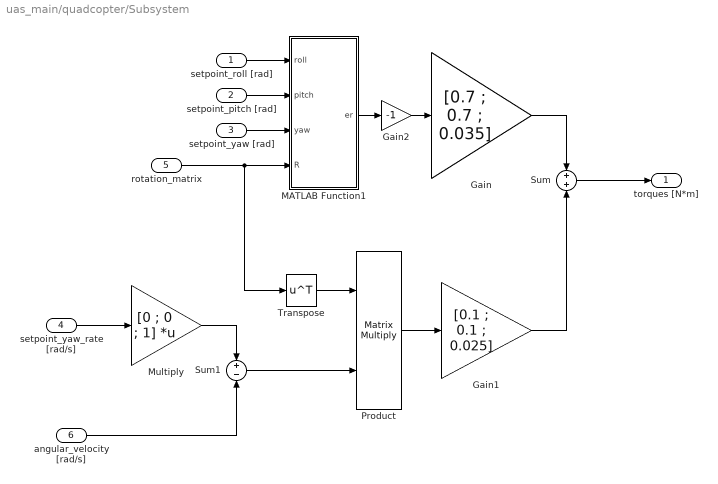
== system uas_main/quadcopter/Subsystem ==
  setpoint_roll [rad] : Inport
  setpoint_pitch [rad] : Inport  Port=2
  setpoint_yaw [rad] : Inport  Port=3
  setpoint_yaw_rate [rad/s] : Inport  Port=4
  rotation_matrix : Inport  Port=5
  angular_velocity [rad/s] : Inport  Port=6
  Gain : Gain  Gain=[0.7 ; 0.7 ; 0.035]
  Gain1 : Gain  Gain=[0.1 ; 0.1 ; 0.025]
  Gain2 : Gain  Gain=-1
  MATLAB Function1 : MATLAB Function  TreatAsAtomicUnit=on
  Multiply : Gain  Gain=[0 ; 0 ; 1]  Multiplication=Matrix(K*u)
  Product : Product  Multiplication=Matrix(*)
  Sum : Sum
  Sum1 : Sum  Inputs=+|-
  Transpose : Math  Operator=transpose  SaturateOnIntegerOverflow=on
  torques [N*m] : Outport
  wires:
  rotation_matrix/1 -> Transpose/1, MATLAB Function1/4(R)
  setpoint_pitch [rad]/1 -> MATLAB Function1/2(pitch)
  Gain2/1 -> Gain/1
  Sum1/1 -> Product/2
  Gain1/1 -> Sum/2
  Multiply/1 -> Sum1/1
  Gain/1 -> Sum/1
  MATLAB Function1/1(er) -> Gain2/1
  setpoint_roll [rad]/1 -> MATLAB Function1/1(roll)
  setpoint_yaw [rad]/1 -> MATLAB Function1/3(yaw)
  Transpose/1 -> Product/1
  setpoint_yaw_rate [rad/s]/1 -> Multiply/1
  Product/1 -> Gain1/1
  angular_velocity [rad/s]/1 -> Sum1/2
  Sum/1 -> torques [N*m]/1

== system uas_main/quadcopter/mixer ==
  In1 : Inport
  Gain5 : Gain  Gain=mix_matrix  Multiplication=Matrix(K*u)
  Saturation : Saturate  UpperLimit=max_rot_velocity^2  LowerLimit=0
  Sqrt : Sqrt  SaturateOnIntegerOverflow=on
  Out1 : Outport
  wires:
  Saturation/1 -> Sqrt/1
  In1/1 -> Gain5/1
  Sqrt/1 -> Out1/1
  Gain5/1 -> Saturation/1
